simulink model "blinky"  (R2020a)
settings: Solver=FixedStepDiscrete  StartTime=0.0  StopTime=10.0  FixedStep=1e-3  RelTol=1e-3
libraries: mbed_lib x3
settings Model: Creator=oh  LastModifiedBy=oh
settings DataIOCC: LimitDataPoints=on  SaveFormat=Array  LoggingToFile=on
settings OptimizationCC: DefaultParameterBehavior=Inlined  EnhancedBackFolding=on  PassReuseOutputArgsAs=Individual arguments  ZeroExternalMemoryAtStartup=off  ZeroInternalMemoryAtStartup=off  OptimizeBlockOrder=speed  DifferentSizesBufferReuse=on  OptimizationCustomize=off  EfficientTunableParamExpr=on
settings DebuggingCC: ParameterTunabilityLossMsg=error  SFUnexpectedBacktrackingDiag=warning  SFNoUnconditionalDefaultTransitionDiag=warning  SFExecutionAtInitializationDiag=none  ArithmeticOperatorsInVariantConditions=warning
settings HardwareCC: ProdBitPerPointer=32  ProdBitPerSizeT=32  ProdBitPerPtrDiffT=32  ProdLargestAtomicInteger=Long  ProdLargestAtomicFloat=Double  ProdWordSize=32  ProdHWDeviceType=ARM Compatible->ARM Cortex
settings ModelReferenceCC: PropagateSignalLabelsOutOfModel=off
settings SFSimCC: SimUseLocalCustomCode=off  MATLABDynamicMemAlloc=off  CustomCodeUndefinedFunction=UseInterfaceOnly
settings RTWCC: Description=MbedTarget (Embedded Target for Embedded Coder)  SystemTargetFile=mbed_ert.tlc  TemplateMakefile=mbed_ert.tmf  RTWUseLocalCustomCode=off  IncludeHyperlinkInReport=on  TargetLang=C++
settings CodeAppCC: ForceParamTrailComments=on  IgnoreCustomStorageClasses=off  OperatorAnnotations=on  SimulinkDataObjDesc=on  SFDataObjDesc=on  InsertBlockDesc=on
settings STFCustomTargetCC: TargetLibSuffix=.a  MultiwordLength=256  GenerateSampleERTMain=on  CombineOutputUpdateFcns=on  ERTCustomFileBanners=on  SupportContinuousTime=off  SupportNonInlinedSFcns=off  RemoveResetFunc=on  MATLABClassNameForMDSCustomization=Simulink.SoftwareTarget.ERTCustomization  ModelStepFunctionPrototypeControlCompliant=on  SystemTargetFile=mbed_ert.tlc
settings ERTTargetCC: GenerateSampleERTMain=on  ParMdlRefBuildCompliant=off  CompOptLevelCompliant=off  ConcurrentExecutionCompliant=off  CPPClassGenCompliant=off  UseToolchainInfoCompliant=off  InlinedParameterPlacement=NonHierarchical  ERTCustomFileTemplate=mbed_ert_file_process.tlc
settings ConfigComp: CovMetricSettings=dw  CovHtmlReporting=on  CovSaveCumulativeToWorkspaceVar=on  CovSaveSingleToWorkspaceVar=on  CovExternalEMLEnable=off

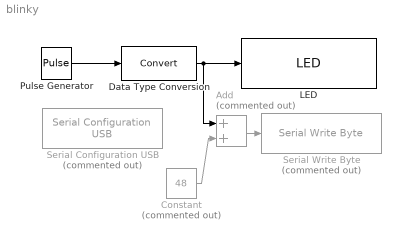
== system blinky ==
  Add : Sum  Commented=on
  Constant : Constant  Commented=on  Value=48  OutDataTypeStr=uint8
  Data Type Conversion : DataTypeConversion
  LED : mbed_lib/GPIO/LED  nLED=1  SampleTime=-1
      settings: SourceProductName=Mbed Target
  Pulse Generator : DiscretePulseGenerator  PulseType=Time based  Period=1  PulseWidth=50
  Serial Configuration USB : mbed_lib/Serial/UART/Serial Configuration USB  Priority=0  Commented=on  BaudRate=115200
      settings: SourceProductName=Mbed Target
  Serial Write Byte : mbed_lib/Serial/UART/Serial Write Byte  Commented=on  SerialPort=USB  SampleTime=0.1
      settings: SourceProductName=Mbed Target
  wires:
  Pulse Generator/1 -> Data Type Conversion/1
  Data Type Conversion/1 -> Add/1, LED/1
  Add/1 -> Serial Write Byte/1
  Constant/1 -> Add/2
